simulink model "combined_vel_estimator_place_holder_name"  (R2024b)
settings: Solver=VariableStepAuto  StartTime=0.0  StopTime=10.0  RelTol=1e-3
settings Model: Creator=lukec  LastModifiedBy=lukec

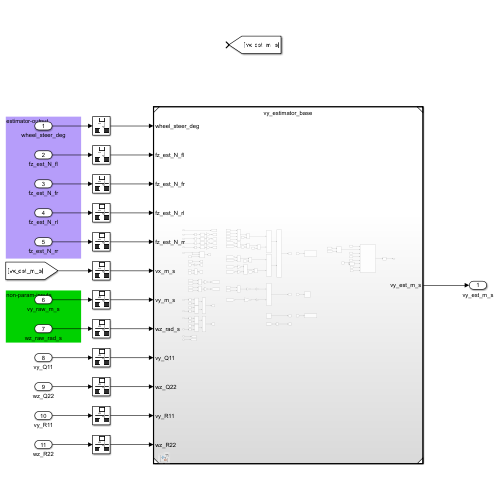
[thumbnail: Simulink's stored preview of the top-level diagram]
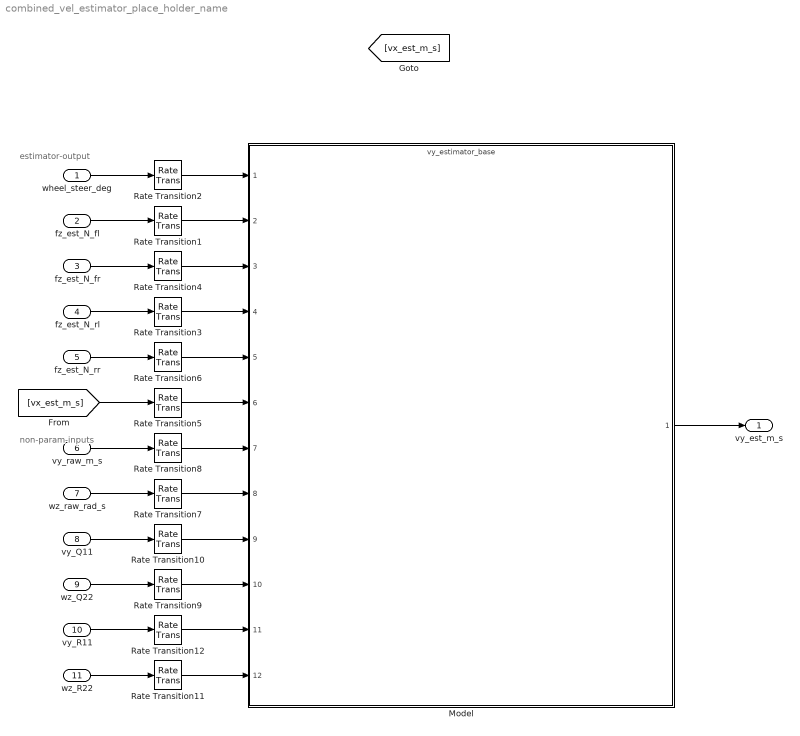
== system combined_vel_estimator_place_holder_name ==
  note: estimator-output
  note: non-param-inputs
  wheel_steer_deg : Inport
  fz_est_N_fl : Inport  Port=2
  fz_est_N_fr : Inport  Port=3
  fz_est_N_rl : Inport  Port=4
  fz_est_N_rr : Inport  Port=5
  vy_raw_m_s : Inport  Port=6
  wz_raw_rad_s : Inport  Port=7
  vy_Q11 : Inport  Port=8
  wz_Q22 : Inport  Port=9
  vy_R11 : Inport  Port=10
  wz_R22 : Inport  Port=11
  Model : ModelReference  ModelNameDialog=vy_estimator_base.slx  SimulationMode=Normal  ModelReferenceVersion=1.5
  Rate Transition{1..12} (12 alike) : RateTransition  OutPortSampleTime=0.004
  vy_est_m_s : Outport
  wires:
  wheel_steer_deg/1 -> Rate Transition2/1
  fz_est_N_fl/1 -> Rate Transition1/1
  fz_est_N_fr/1 -> Rate Transition4/1
  fz_est_N_rl/1 -> Rate Transition3/1
  fz_est_N_rr/1 -> Rate Transition6/1
  [vx_est_m_s] -> Rate Transition5/1
  vy_raw_m_s/1 -> Rate Transition8/1
  wz_raw_rad_s/1 -> Rate Transition7/1
  vy_Q11/1 -> Rate Transition10/1
  wz_Q22/1 -> Rate Transition9/1
  vy_R11/1 -> Rate Transition12/1
  wz_R22/1 -> Rate Transition11/1
  Rate Transition2/1 -> Model/1
  Rate Transition1/1 -> Model/2
  Rate Transition4/1 -> Model/3
  Rate Transition3/1 -> Model/4
  Rate Transition6/1 -> Model/5
  Rate Transition7/1 -> Model/8
  Rate Transition5/1 -> Model/6
  Rate Transition8/1 -> Model/7
  Rate Transition12/1 -> Model/11
  Rate Transition10/1 -> Model/9
  Rate Transition9/1 -> Model/10
  Rate Transition11/1 -> Model/12
  Model/1 -> vy_est_m_s/1
